simulink model "test_rfdc_yb"  (R2018b)
settings: Solver=VariableStepAuto  StartTime=0.0  StopTime=10.0  RelTol=1e-3
libraries: xbsIndex_r4 x5, xps_library x1
settings Model: Creator=mcb  LastModifiedBy=mcb

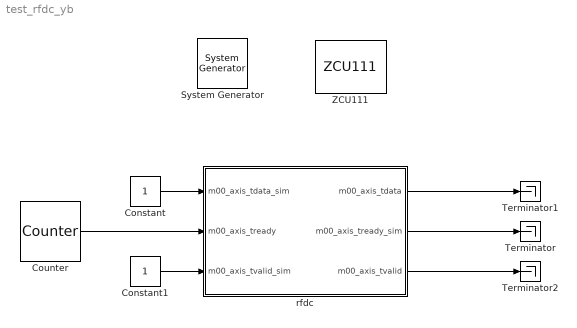
== system test_rfdc_yb ==
  " System Generator" : xbsIndex_r4/ System Generator  Tag=genX  xilinxfamily=zynquplusRFSOC  part=xczu28dr  speed=-2-e  package=ffvg1517  synthesis_tool=XST  clock_wrapper=Clock Enables  directory=/home/mcb/git/casper-astro/mlib_devel/workspace/rfdc-port/rfdc_yb/sysgen  proj_type=Vivado  Synth_file=Vivado Synthesis Defaults  Impl_file=Vivado Implementation Defaults  testbench=off  simulink_period=1  sysclk_period=10  dcm_input_clock_period=10  incr_netlist=off  trim_vbits=Everywhere in SubSystem  dbl_ovrd=According to Block Masks  core_generation=According to Block Masks  run_coregen=off  deprecated_control=off  eval_field=0  block_type=sysgen
  Constant : Constant
  Constant1 : Constant
  Counter : xbsIndex_r4/Counter  cnt_type=Free Running  cnt_to=Inf  operation=Up  start_count=0  cnt_by_val=1  arith_type=Unsigned  n_bits=1  bin_pt=0  load_pin=off  rst=off  en=off  explicit_period=on  period=1  use_behavioral_HDL=off  implementation=Fabric  dbl_ovrd=off  block_type=counter
  Terminator : Terminator
  Terminator1 : Terminator
  Terminator2 : Terminator
  ZCU111 : xps_library/Platforms/ZCU111  Tag=xps:xsg  hw_sys=ZCU111:xczu28dr  clk_src=sys_clk  clk_rate=100  sample_period=1  synthesis_tool=XST
      settings: SourceProductName=CASPER XPS Blockset
  rfdc : Subsystem  Tag=xps:rfdc  mask(rfdc){tile_224_adc0_enable=on, tile_224_adc0_sample_per_cycle=1, tile_224_adc1_enable=on}
      mask prompts: tile_224_adc0_enable "Enable ADC"; tile_224_adc0_sample_per_cycle "Samples per AXI4-Stream Cycle"; tile_224_adc1_enable "Enable ADC"
      mask help: Xilinx RF Data Converter Yellow Block
      mask init:
      | %rfdc_init(gcb);
      mask Help: This is the CASPER "yellow block" for the Xilinx RFSoC
      mask TypeOptions tile_224_adc0_sample_per_cycle: 1 | 2 | 3 | 4 | 5 | 6 | 7 | 8
      mask DialogControl adc_tile_224 Prompt: ADC Tile 224
      mask DialogControl pll_clocking_config_224 Prompt: PLL and Clocking
      mask DialogControl tile_224_adc0 Prompt: ADC 0
      mask DialogControl tile_224_adc0_data_settings Prompt: Data Settings
      mask DialogControl tile_224_adc1 Prompt: ADC 1
      mask DialogControl adc_tile_225 Prompt: ADC Tile 225
      mask DialogControl adc_tile_226 Prompt: ADC Tile 226
      mask DialogControl adc_tile_227 Prompt: ADC Tile 227
  wires:
  Constant/1 -> rfdc/1(m00_axis_tdata_sim)
  Constant1/1 -> rfdc/3(m00_axis_tvalid_sim)
  Counter/1 -> rfdc/2(m00_axis_tready)
  rfdc/2(m00_axis_tready_sim) -> Terminator/1
  rfdc/1(m00_axis_tdata) -> Terminator1/1
  rfdc/3(m00_axis_tvalid) -> Terminator2/1

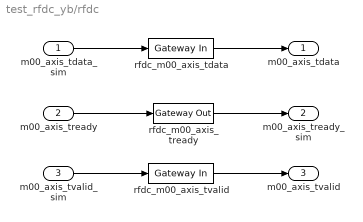
== system test_rfdc_yb/rfdc ==
  m00_axis_tdata_sim : Inport
  m00_axis_tready : Inport  Port=2
  m00_axis_tvalid_sim : Inport  Port=3
  rfdc_m00_axis_tdata : xbsIndex_r4/Gateway In  gui_display_data_type=Fixed-point  arith_type="Signed  (2's comp)"  n_bits=16  bin_pt=14  preci_type=Single  exp_width=8  frac_width=24  rows=1  columns=1  quantization="Round  (unbiased: +/- Inf)"  overflow=Saturate  period=1  UseAsADC=off  ADCChannel='1'  interface=None  automatic_assignment=on  address_offset=hex2dec('00')  intf_name=''  intf_description=''  default_value=0  timing_constraint=None  locs_specified=off  LOCs={}  io_standard={}  inherit_from_input=off  hdl_port=on  dbl_ovrd=off  block_type=gatewayin
  rfdc_m00_axis_tready : xbsIndex_r4/Gateway Out  inherit_from_input=off  hdl_port=on  rows=1  columns=1  UseAsDAC=off  DACChannel='1'  interface=None  automatic_assignment=on  address_offset=hex2dec('00')  intf_name=''  intf_description=''  timing_constraint=None  locs_specified=off  LOCs={}  io_standard={}  block_type=gatewayout
  rfdc_m00_axis_tvalid : xbsIndex_r4/Gateway In  gui_display_data_type=Fixed-point  arith_type="Signed  (2's comp)"  n_bits=16  bin_pt=14  preci_type=Single  exp_width=8  frac_width=24  rows=1  columns=1  quantization="Round  (unbiased: +/- Inf)"  overflow=Saturate  period=1  UseAsADC=off  ADCChannel='1'  interface=None  automatic_assignment=on  address_offset=hex2dec('00')  intf_name=''  intf_description=''  default_value=0  timing_constraint=None  locs_specified=off  LOCs={}  io_standard={}  inherit_from_input=off  hdl_port=on  dbl_ovrd=off  block_type=gatewayin
  m00_axis_tdata : Outport
  m00_axis_tready_sim : Outport  Port=2
  m00_axis_tvalid : Outport  Port=3
  wires:
  m00_axis_tdata_sim/1 -> rfdc_m00_axis_tdata/1
  rfdc_m00_axis_tdata/1 -> m00_axis_tdata/1
  rfdc_m00_axis_tready/1 -> m00_axis_tready_sim/1
  rfdc_m00_axis_tvalid/1 -> m00_axis_tvalid/1
  m00_axis_tready/1 -> rfdc_m00_axis_tready/1
  m00_axis_tvalid_sim/1 -> rfdc_m00_axis_tvalid/1
